simulink model "turbo_code_punc"  (Simulink 6.5)
settings: Solver=VariableStepDiscrete  StartTime=0.0  StopTime=50  FixedStep=Auto  RelTol=1e-3
PostLoadFcn:
  | turbo_code_punc_setup;
undefined symbols (not defined in the file or in its folder): Iter, Len, Max, Variance
libraries: commsequence2 x6, commblkintrlv2 x6, commcnvcod2 x4, commchan3 x1, commrandsrc2 x1, dspbuff3 x1, commsink2 x1, dspstat3 x1, dspsrcs4 x1, dspindex x1, dspsigops x1, simulink_obsolete x1
Description:
  | a turbo code
  | 1/2 code rate, with puncturing
  | 
  | generator polynomials
  | G =[1 1 1 1 1
  |         1 0 0 0 1]
  | 
  | Reference:  Digital Communications, 2nd edition, B. Sklar,
  |                         2001, Prentice Hall
  |                         pp. 496-497.
settings Model: Creator=In Soo Ahn  LastModifiedBy=isa
settings Model: ModifiedHistory=|
  | Your comments and suggestions are welcome.
  | isa@bradley.edu
settings SolverCC: ConsecutiveZCsStepRelTol=1*128*eps
settings DebuggingCC: DiscreteInheritContinuousMsg=error  MultiTaskDSMMsg=warning  MultiTaskCondExecSysMsg=none
settings RTWCC: IncludeERTFirstTime=on

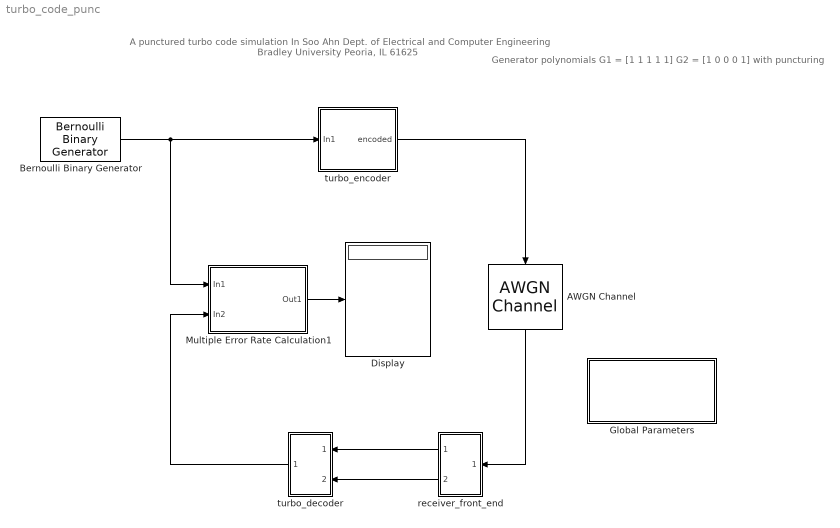
== system turbo_code_punc ==
  note: A punctured turbo code simulation
      | In Soo Ahn
      | Dept. of Electrical and Computer Engineering
      | Bradley University
      | Peoria, IL 61625
  note: Generator polynomials
      | G1 = [1 1 1 1 1]
      | G2 = [1 0 0 0 1]
      | with puncturing
  AWGN Channel : commchan3/AWGN Channel  Orientation=down  SystemSampleTime=-1  seed=1  noiseMode=Variance from mask  EbNodB=2  EsNodB=10  SNRdB=10  bitsPerSym=2  Ps=1  Tsym=Iter/Len  variance=Variance
  Bernoulli Binary Generator : commrandsrc2/Bernoulli Binary Generator  DialogController=commDDGCreate  DialogControllerArgs=DataTag0  SystemSampleTime=-1  P=0.5  seed=61  Ts=1  frameBased=on  sampPerFrame=Len  orient=off  outDataType=boolean
  Display : Display
  Global Parameters : Subsystem  mask(Global Parameters){EbNodB=2, Len=256*256, Iter=5, Seed=54123}
      mask prompts: EbNodB "Eb/No in dB:"; Len "Block size:"; Iter "Number of iterations:"
      mask help: Load global parameters in MATLAB workspace.
      mask init:
      | turbo_code_punc_setup;
      mask CallbackString: turbo_code_setup;|turbo_code_setup|turbo_code_setup;|turbo_code_setup;
      mask Display:
      | disp(['Eb/No ' num2str(EbNodB,'%3.1f') 'dB'
      | sprintf('\n') 'Block size   ' num2str(Len,'%7.0f')
      | sprintf('\n') 'Iterations   ' num2str(Iter,'%3.0f')
      | sprintf('\n') 'Seed   ' num2str(Seed,'%7.0f')])
  Multiple Error Rate Calculation1 : Subsystem
      mask Display: disp('Multiple\nIteration\nError Rate\nCalculation')
  receiver_front_end : Subsystem  Orientation=left
  turbo_decoder : Subsystem  Orientation=left
  turbo_encoder : Subsystem
  wires:
  Multiple Error Rate Calculation1/1(Out1) -> Display/1
  turbo_decoder/1(Out1) -> Multiple Error Rate Calculation1/2(In2)
  Bernoulli Binary Generator/1 -> turbo_encoder/1(In1), Multiple Error Rate Calculation1/1(In1)
  receiver_front_end/1(Out1) -> turbo_decoder/1(In1)
  receiver_front_end/2(Out2) -> turbo_decoder/2(In2)
  turbo_encoder/1(encoded) -> AWGN Channel/1
  AWGN Channel/1 -> receiver_front_end/1(In1)

== system turbo_code_punc/Global Parameters ==

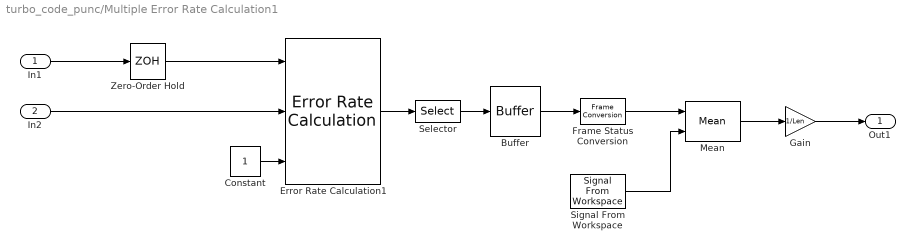
== system turbo_code_punc/Multiple Error Rate Calculation1 ==
  In1 : Inport
  In2 : Inport  Port=2
  Buffer : dspbuff3/Buffer  N=Iter  V=0  ic=0
  Constant : Constant  Value=1  OutDataType=sfix(16)  ConRadixGroup=Use specified scaling  OutScaling=2^0  SampleTime=inf  FramePeriod=inf
  Error Rate Calculation1 : commsink2/Error Rate Calculation  N=0  st_delay=0  cp_mode=Entire frame  subframe=[]  PMode=Port  WsName=ErrorVec1  RsMode2=on  stop=off  numErr=100  maxBits=1e6
  Frame Status Conversion : FrameConversion  OutFrame=Sample based
  Gain : Gain  Gain=1/Len  SaturateOnIntegerOverflow=on
  Mean : dspstat3/Mean  DialogController=dspDDGCreate  DialogControllerArgs=DataTag1  run=on  reset_popup=Non-zero sample  roundingMode=Floor  overflowMode=off
  Selector : Selector  InputType=Vector  ElementSrc=Internal  Elements=2  RowSrc=Internal  Rows=1  ColumnSrc=Internal  Columns=1  InputPortWidth=3  IndexIsStartValue=off
  Signal From Workspace : dspsrcs4/Signal From Workspace  SystemSampleTime=-1  X=[1 1]  Ts=Iter  nsamps=1  OutputAfterFinalValue=Setting to zero  ignoreOrWarnInputAndFrameLengths=off
  Zero-Order Hold : ZeroOrderHold
  Out1 : Outport
  wires:
  In1/1 -> Zero-Order Hold/1
  Error Rate Calculation1/1 -> Selector/1
  Selector/1 -> Buffer/1
  In2/1 -> Error Rate Calculation1/2
  Buffer/1 -> Frame Status Conversion/1
  Frame Status Conversion/1 -> Mean/1
  Zero-Order Hold/1 -> Error Rate Calculation1/1
  Constant/1 -> Error Rate Calculation1/3
  Mean/1 -> Gain/1
  Gain/1 -> Out1/1
  Signal From Workspace/1 -> Mean/2

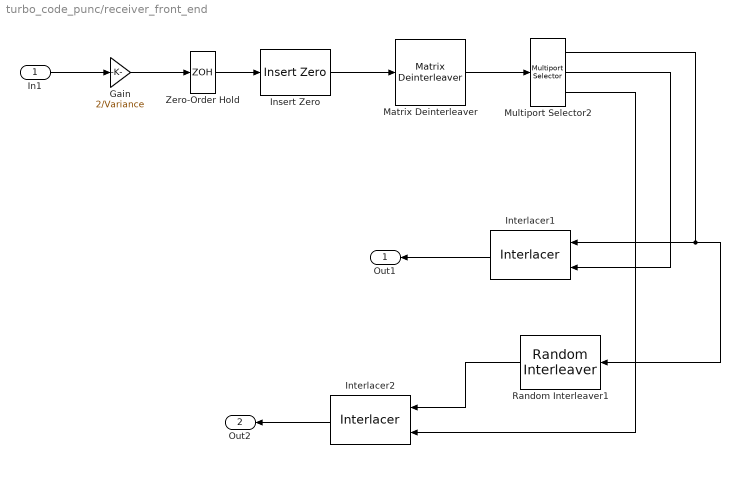
== system turbo_code_punc/receiver_front_end ==
  In1 : Inport
  Gain : Gain  Gain=2/Variance  SampleTime=1
  Insert Zero : commsequence2/Insert Zero  insertZeroVector=[1 1 0 1 0 1].'
  Interlacer1 : commsequence2/Interlacer  Orientation=left
  Interlacer2 : commsequence2/Interlacer  Orientation=left
  Matrix Deinterleaver : commblkintrlv2/Matrix Deinterleaver  SystemSampleTime=-1  Nrows=3  Ncols=Len
  Multiport Selector2 : dspindex/Multiport Selector  rowsOrCols=Rows  idxCellArray={1:Len, Len+1:2*Len, 2*Len+1:3*Len}  idxErrMode=Clip Index
  Random Interleaver1 : commblkintrlv2/Random Interleaver  Orientation=left  SystemSampleTime=-1  N=Len  seed=Seed
  Zero-Order Hold : ZeroOrderHold  SampleTime=Iter
  Out1 : Outport  Orientation=left
  Out2 : Outport  Orientation=left  Port=2
  wires:
  Multiport Selector2/1 -> Interlacer1/1, Random Interleaver1/1
  Multiport Selector2/2 -> Interlacer1/2
  Random Interleaver1/1 -> Interlacer2/1
  Multiport Selector2/3 -> Interlacer2/2
  Zero-Order Hold/1 -> Insert Zero/1
  In1/1 -> Gain/1
  Interlacer1/1 -> Out1/1
  Interlacer2/1 -> Out2/1
  Matrix Deinterleaver/1 -> Multiport Selector2/1
  Insert Zero/1 -> Matrix Deinterleaver/1
  Gain/1 -> Zero-Order Hold/1

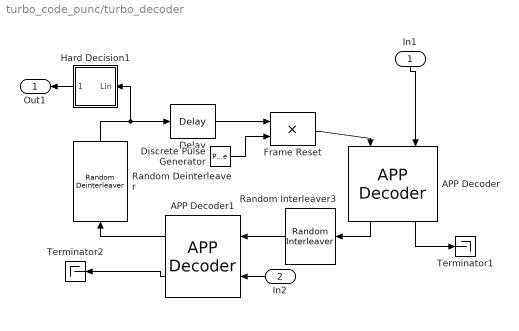
== system turbo_code_punc/turbo_decoder ==
  In1 : Inport  Orientation=down
  In2 : Inport  Orientation=left  Port=2
  APP Decoder : commcnvcod2/APP Decoder  Orientation=down  trellis=trellis  termMethod=Truncated  algorithm=Max*  maxStarNumScaleBits=3
  APP Decoder1 : commcnvcod2/APP Decoder  Orientation=left  trellis=trellis  termMethod=Truncated  algorithm=Max*  maxStarNumScaleBits=3
  Delay : dspsigops/Delay  dly_unit=Samples  delay=Len  ic_detail=off  dif_ic_for_ch=off  dif_ic_for_dly=off  ic=0  reset_popup=None
  Discrete Pulse Generator : DiscretePulseGenerator  Period=Iter  PulseWidth=Iter-1  PhaseDelay=1
  Frame Reset : Product  SaturateOnIntegerOverflow=on  InputSameDT=on
  Hard Decision1 : Subsystem  Orientation=left
      mask Type: Hard Decision
      mask Description: Likelihood to binary transformation.
  Random Deinterleaver : commblkintrlv2/Random Deinterleaver  Orientation=up  SystemSampleTime=-1  N=Len  seed=Seed
  Random Interleaver3 : commblkintrlv2/Random Interleaver  Orientation=left  SystemSampleTime=-1  N=Len  seed=Seed
  Terminator1 : Terminator
  Terminator2 : Terminator
  Out1 : Outport  Orientation=left
  wires:
  APP Decoder1/1 -> Random Deinterleaver/1
  APP Decoder/2 -> Terminator1/1
  APP Decoder1/2 -> Terminator2/1
  Random Deinterleaver/1 -> Delay/1, Hard Decision1/1(Lin)
  Random Interleaver3/1 -> APP Decoder1/1
  APP Decoder/1 -> Random Interleaver3/1
  Frame Reset/1 -> APP Decoder/1
  Delay/1 -> Frame Reset/1
  Discrete Pulse Generator/1 -> Frame Reset/2
  Hard Decision1/1(0/1) -> Out1/1
  In1/1 -> APP Decoder/2
  In2/1 -> APP Decoder1/2

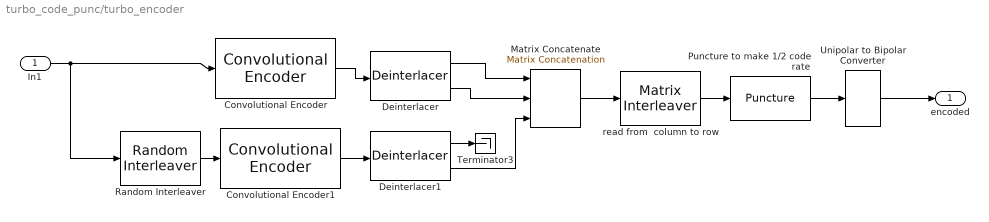
== system turbo_code_punc/turbo_encoder ==
  In1 : Inport
  Convolutional Encoder : commcnvcod2/Convolutional Encoder  trellis=trellis  opMode=Continuous  usePuncVector=off  punctureVector=[ 1 1 0 1 0 1]'  reset=Unused parameter value
  Convolutional Encoder1 : commcnvcod2/Convolutional Encoder  trellis=trellis  opMode=Truncated (reset every frame)  usePuncVector=off  punctureVector=[ 1 1 0 1 0 1]'  reset=Unused parameter value
  Deinterlacer : commsequence2/Deinterlacer
  Deinterlacer1 : commsequence2/Deinterlacer
  Matrix Concatenate : simulink_obsolete/Matrix Concatenation  numInports=3  catMethod=Vertical
  Puncture to make 1/2 code rate : commsequence2/Puncture  punctureVector=[1 1 0 1 0 1].'
  Random Interleaver : commblkintrlv2/Random Interleaver  SystemSampleTime=-1  N=Len  seed=Seed
  Terminator3 : Terminator
  Unipolar to Bipolar Converter : commutil2/Unipolar to Bipolar Converter  SystemSampleTime=-1  M=2  polarity=Positive  dataType=double
  read from  column to row : commblkintrlv2/Matrix Interleaver  SystemSampleTime=-1  Nrows=3  Ncols=Len
  encoded : Outport
  wires:
  In1/1 -> Convolutional Encoder/1, Random Interleaver/1
  Unipolar to Bipolar Converter/1 -> encoded/1
  Random Interleaver/1 -> Convolutional Encoder1/1
  Convolutional Encoder/1 -> Deinterlacer/1
  Convolutional Encoder1/1 -> Deinterlacer1/1
  Deinterlacer1/1 -> Terminator3/1
  Deinterlacer/1 -> Matrix Concatenate/1
  Deinterlacer/2 -> Matrix Concatenate/2
  Deinterlacer1/2 -> Matrix Concatenate/3
  read from  column to row/1 -> Puncture to make 1/2 code rate/1
  Matrix Concatenate/1 -> read from  column to row/1
  Puncture to make 1/2 code rate/1 -> Unipolar to Bipolar Converter/1

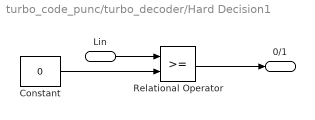
== system turbo_code_punc/turbo_decoder/Hard Decision1 ==
  Lin : Inport
  Constant : Constant  Value=0  OutDataType=sfix(16)  ConRadixGroup=Use specified scaling  OutScaling=2^0  SampleTime=inf  FramePeriod=inf
  Relational Operator : RelationalOperator  InputSameDT=on
  0/1 : Outport
  wires:
  Constant/1 -> Relational Operator/2
  Lin/1 -> Relational Operator/1
  Relational Operator/1 -> 0/1/1
